simulink model "MAJOR_PROJECT_FINAL"  (R2023b)
settings: Solver=VariableStepAuto  StartTime=0.0  StopTime=inf  FixedStep=1  RelTol=1e-3
libraries: spsRMSLib x8, spsCurrentMeasurementLib x4, spsVoltageMeasurementLib x4, spsPowerLib x4, spsBreakerLib x3, spsSeriesRLCBranchLib x3, spsACVoltageSourceLib x1, spsPLLLib x1, sps_lib x1
settings Model: Creator=bhavikg27  LastModifiedBy=bhavikg27

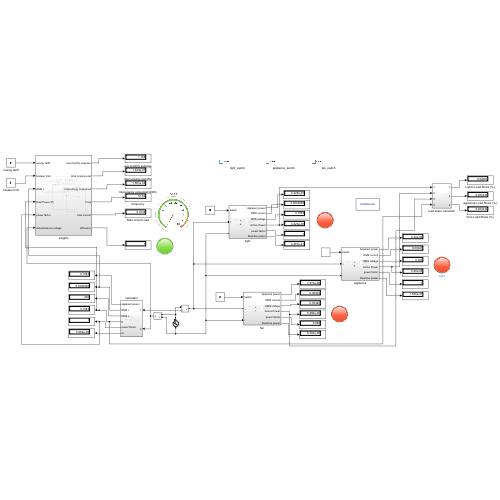
[thumbnail: Simulink's stored preview of the top-level diagram]
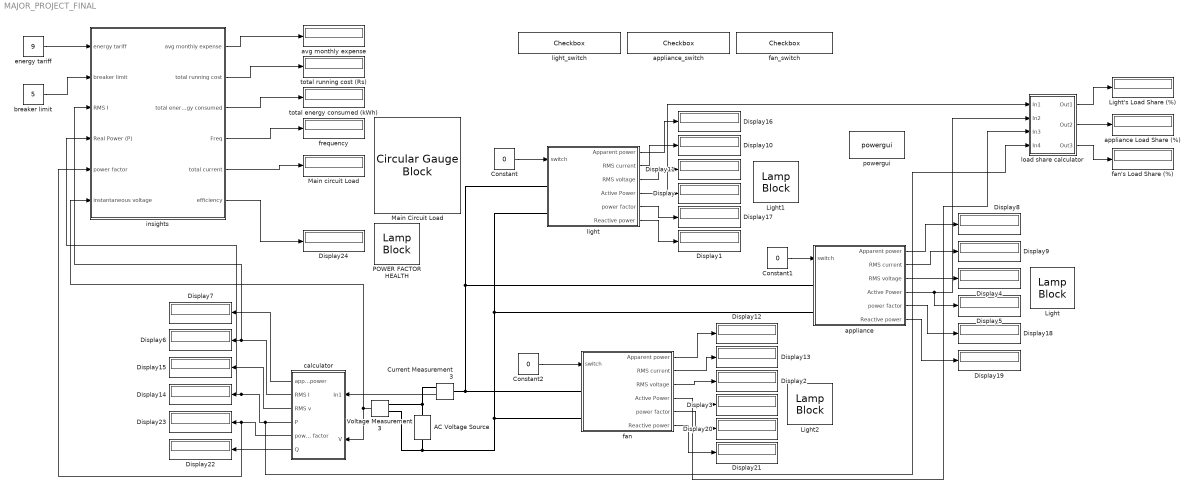
== system MAJOR_PROJECT_FINAL ==
  AC Voltage Source : spsACVoltageSourceLib/AC Voltage Source  Amplitude=325.27  Phase=0  Frequency=50  SampleTime=0  Measurements=None  BusType=swing  Pref=10e3  Qref=0  Qmin=-inf  Qmax=+inf
  Constant : Constant  Value=0
  Constant1 : Constant  Value=0
  Constant2 : Constant  Value=0
  Current Measurement3 : spsCurrentMeasurementLib/Current Measurement  PhasorSimulation=off  OutputType=Complex  PSBequivalent=0
  Display{,1..24} (25 alike) : Display
  Light : LampBlock  LabelPosition=Hide
  Light's Load Share (%) : Display
  Light1 : LampBlock  LabelPosition=Hide
  Light2 : LampBlock  LabelPosition=Hide
  Main Circuit Load : CircularGaugeBlock
  Main circuit Load : Display
  POWER FACTOR HEALTH : LampBlock  LabelPosition=Hide
  Voltage Measurement3 : spsVoltageMeasurementLib/Voltage Measurement  PhasorSimulation=off  OutputType=Complex  PSBequivalent=0
  appliance : Subsystem
  appliance Load Share (%) : Display
  appliance_switch : Checkbox  LabelPosition=Hide  ShowInitialText=on
  avg monthly expense : Display
  breaker limit : Constant  Value=5
  calculator : Subsystem
  energy tariff : Constant  Value=9
  fan : Subsystem
  fan's Load Share (%) : Display
  fan_switch : Checkbox  LabelPosition=Hide  ShowInitialText=on
  frequency : Display
  insights : Subsystem
  light : Subsystem
  light_switch : Checkbox  LabelPosition=Hide  ShowInitialText=on
  load share calculator : Subsystem
  powergui : sps_lib/powergui  Priority=1  SimulationMode=Continuous  SampleTime=50e-6  frequency=60  Iterations=50  frequencyindice=50  Pbase=100e6  ErrMax=1e-4  UnitsV=kV  UnitsW=MW  buscounter=0  FunctionMessages=off  echomessages=off  EnableUseOfTLC=off  CurrentSourceSwitches=off  DisableSnubberDevices=off  DisableRonSwitches=off  DisableVfSwitches=off  DisplayEquations=off  AutomaticDiscreteSolvers=off  SolverType=Tustin/Backward Euler (TBE)  Interpol=off  ExternalGateDelay=off  methode=off  Ts=100  x0status=blocks  SPID=on  SwTol=0  HookPort=off  NonlinearTolerance=1e-4  nMaxIteration=100  ContinueOnMaxIteration=off  RestoreLinks=warning  ResistiveCurrentMeasurement=off  Frange=[0:2:500]  Ylog=off  Xlog=on  ShowGrid=off  save=off  variable=ZData  structure=0  ZoomFFT=off  StartTime=0.0  cycles=1  DisplayStyle=1  fundamental=60  FreqAxis=off  MaxFrequency=1000  frequencyindicesteady=1  RmsSteady=1  display=off
  total energy consumed (kWh) : Display
  total running cost (Rs) : Display
  wires:
  Constant1/1 -> appliance/1(switch)
  Constant2/1 -> fan/1(switch)
  Constant/1 -> light/1(switch)
  light/2(RMS current) -> Display10/1
  light/3(RMS voltage) -> Display11/1
  light/4(Active Power) -> load share calculator/1(In1), Display/1
  light/6(Reactive power) -> Display1/1
  light/1(Apparent power) -> Display16/1
  light/5(power factor) -> Display17/1
  fan/1(Apparent power) -> Display12/1
  fan/3(RMS voltage) -> Display2/1
  fan/4(Active Power) -> load share calculator/3(In3), Display3/1
  fan/6(Reactive power) -> Display21/1
  fan/5(power factor) -> Display20/1
  appliance/1(Apparent power) -> Display8/1
  appliance/2(RMS current) -> Display9/1
  appliance/3(RMS voltage) -> Display4/1
  appliance/4(Active Power) -> load share calculator/2(In2), Display5/1
  appliance/5(power factor) -> Display18/1
  appliance/6(Reactive power) -> Display19/1
  fan/2(RMS current) -> Display13/1
  Voltage Measurement3/1 -> calculator/2(V), insights/6(instantaneous voltage)
  Current Measurement3/1 -> calculator/1(In1)
  calculator/1(apparant power) -> Display7/1
  calculator/2(RMS I) -> insights/3(RMS I), Display6/1
  calculator/3(RMS v) -> Display15/1
  calculator/4(P) -> load share calculator/4(In4), insights/4(Real Power (P)), Display14/1
  calculator/5(power factor) -> insights/5(power factor), Display23/1
  calculator/6(Q) -> Display22/1
  load share calculator/1(Out1) -> Light's Load Share (%)/1
  load share calculator/2(Out2) -> appliance Load Share (%)/1
  load share calculator/3(Out3) -> fan's Load Share (%)/1
  energy tariff/1 -> insights/1(energy tariff)
  breaker limit/1 -> insights/2(breaker limit)
  insights/1(avg monthly expense) -> avg monthly expense/1
  insights/2(total running cost) -> total running cost (Rs)/1
  insights/3(total energy consumed) -> total energy consumed (kWh)/1
  insights/4(Freq) -> frequency/1
  insights/5(total current) -> Main circuit Load/1
  insights/6(efficiency) -> Display24/1
  connections:
  Voltage Measurement3/LConn1 -- AC Voltage Source/LConn1 -- light/LConn2 -- appliance/LConn2 -- fan/LConn2
  Current Measurement3/RConn1 -- Voltage Measurement3/LConn2 -- AC Voltage Source/RConn1
  Current Measurement3/LConn1 -- fan/LConn1 -- light/LConn1 -- appliance/LConn1

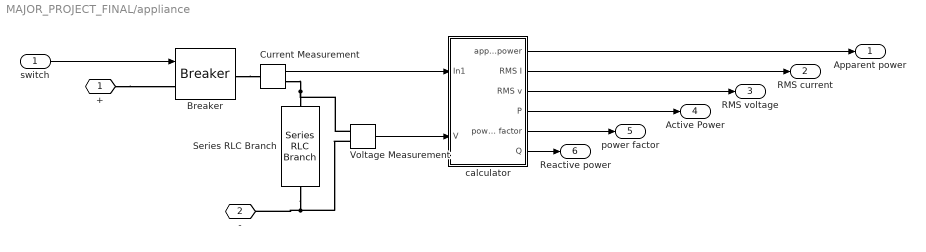
== system MAJOR_PROJECT_FINAL/appliance ==
  switch : Inport
  Breaker : spsBreakerLib/Breaker  InitialState=0  SwitchingTimes="[1/60  5/60]"  External=on  BreakerResistance=0.01  SnubberResistance=1e6  SnubberCapacitance=inf  Measurements=None  MoreParameters=on  NoBreakLoop=off
  Current Measurement : spsCurrentMeasurementLib/Current Measurement  PhasorSimulation=off  OutputType=Complex  PSBequivalent=0
  Series RLC Branch : spsSeriesRLCBranchLib/Series RLC Branch  LConnTagsString=__new0  RConnTagsString=__new0  BranchType=R  Resistance=100  Inductance=1e-3  SetiL0=off  InitialCurrent=0  Capacitance=1e-6  Setx0=off  InitialVoltage=0  Measurements=None
  Voltage Measurement : spsVoltageMeasurementLib/Voltage Measurement  PhasorSimulation=off  OutputType=Complex  PSBequivalent=0
  calculator : Subsystem
  + : PMIOPort  Side=Left
  - : PMIOPort  Port=2  Side=Left
  Apparent power : Outport
  RMS current : Outport  Port=2
  RMS voltage : Outport  Port=3
  Active Power : Outport  Port=4
  power factor : Outport  Port=5
  Reactive power : Outport  Port=6
  wires:
  switch/1 -> Breaker/1
  calculator/5(power factor) -> power factor/1
  calculator/6(Q) -> Reactive power/1
  calculator/4(P) -> Active Power/1
  calculator/2(RMS I) -> RMS current/1
  Voltage Measurement/1 -> calculator/2(V)
  Current Measurement/1 -> calculator/1(In1)
  calculator/1(apparant power) -> Apparent power/1
  calculator/3(RMS v) -> RMS voltage/1
  connections:
  +/RConn1 -- Breaker/LConn1
  Breaker/RConn1 -- Current Measurement/LConn1
  Series RLC Branch/RConn1 -- Voltage Measurement/LConn2 -- -/RConn1
  Current Measurement/RConn1 -- Voltage Measurement/LConn1 -- Series RLC Branch/LConn1

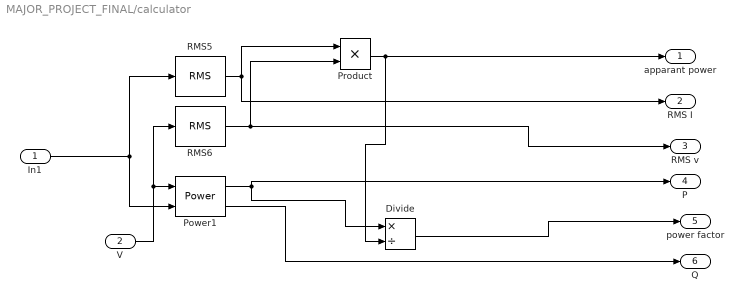
== system MAJOR_PROJECT_FINAL/calculator ==
  In1 : Inport
  V : Inport  Port=2
  Divide : Product  Inputs=*/
  Power1 : spsPowerLib/Power  Freq=50  Vinit=[1, 0]  Iinit=[1, 0]  Ts=0
  Product : Product
  RMS5 : spsRMSLib/RMS  TrueRMS=on  Freq=50  RMSInit=120  Ts=0
  RMS6 : spsRMSLib/RMS  TrueRMS=on  Freq=50  RMSInit=120  Ts=0
  apparant power : Outport
  RMS I : Outport  Port=2
  RMS v : Outport  Port=3
  P : Outport  Port=4
  power factor : Outport  Port=5
  Q : Outport  Port=6
  wires:
  V/1 -> RMS6/1, Power1/1
  In1/1 -> Power1/2, RMS5/1
  RMS5/1 -> RMS I/1, Product/1
  RMS6/1 -> RMS v/1, Product/2
  Power1/1 -> P/1, Divide/1
  Product/1 -> apparant power/1, Divide/2
  Divide/1 -> power factor/1
  Power1/2 -> Q/1

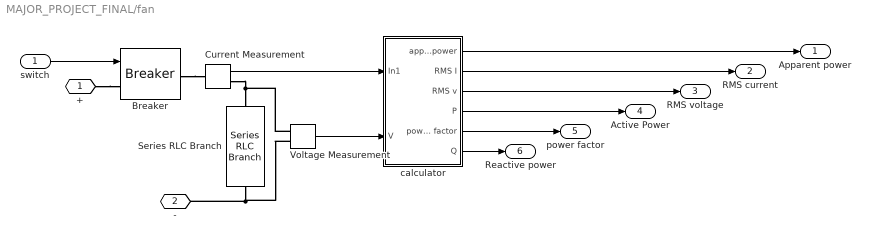
== system MAJOR_PROJECT_FINAL/fan ==
  switch : Inport
  Breaker : spsBreakerLib/Breaker  InitialState=0  SwitchingTimes="[1/60  5/60]"  External=on  BreakerResistance=0.01  SnubberResistance=1e6  SnubberCapacitance=inf  Measurements=None  MoreParameters=on  NoBreakLoop=off
  Current Measurement : spsCurrentMeasurementLib/Current Measurement  PhasorSimulation=off  OutputType=Complex  PSBequivalent=0
  Series RLC Branch : spsSeriesRLCBranchLib/Series RLC Branch  LConnTagsString=__new0  RConnTagsString=__new0  BranchType=RL  Resistance=100  Inductance=0.3  SetiL0=off  InitialCurrent=0  Capacitance=1e-6  Setx0=off  InitialVoltage=0  Measurements=None
  Voltage Measurement : spsVoltageMeasurementLib/Voltage Measurement  PhasorSimulation=off  OutputType=Complex  PSBequivalent=0
  calculator : Subsystem
  + : PMIOPort  Side=Left
  - : PMIOPort  Port=2  Side=Left
  Apparent power : Outport
  RMS current : Outport  Port=2
  RMS voltage : Outport  Port=3
  Active Power : Outport  Port=4
  power factor : Outport  Port=5
  Reactive power : Outport  Port=6
  wires:
  switch/1 -> Breaker/1
  calculator/5(power factor) -> power factor/1
  calculator/6(Q) -> Reactive power/1
  calculator/4(P) -> Active Power/1
  calculator/2(RMS I) -> RMS current/1
  Voltage Measurement/1 -> calculator/2(V)
  Current Measurement/1 -> calculator/1(In1)
  calculator/1(apparant power) -> Apparent power/1
  calculator/3(RMS v) -> RMS voltage/1
  connections:
  +/RConn1 -- Breaker/LConn1
  Breaker/RConn1 -- Current Measurement/LConn1
  Series RLC Branch/RConn1 -- -/RConn1 -- Voltage Measurement/LConn2
  Current Measurement/RConn1 -- Voltage Measurement/LConn1 -- Series RLC Branch/LConn1

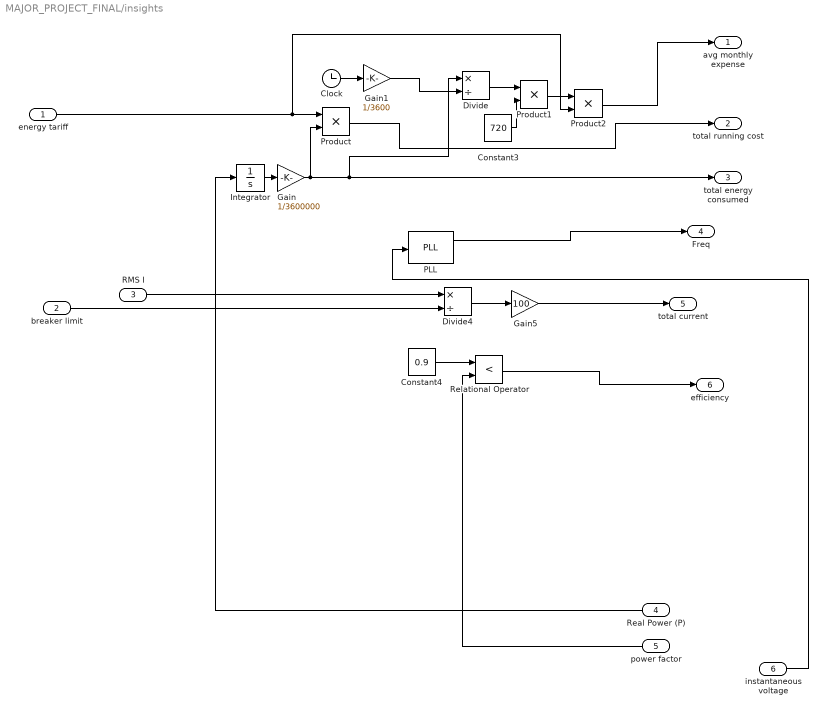
== system MAJOR_PROJECT_FINAL/insights ==
  energy tariff : Inport
  breaker limit : Inport  Port=2
  RMS I : Inport  Port=3
  Real Power (P) : Inport  Port=4
  power factor : Inport  Port=5
  instantaneous voltage : Inport  Port=6
  Clock : Clock
  Constant3 : Constant  Value=720
  Constant4 : Constant  Value=0.9
  Divide : Product  Inputs=*/
  Divide4 : Product  Inputs=*/
  Gain : Gain  Gain=1/3600000
  Gain1 : Gain  Gain=1/3600
  Gain5 : Gain  Gain=100
  Integrator : Integrator
  PLL : spsPLLLib/PLL  Fmin=45  Par_Init=[0, 60]  ParK=[180, 3200, 1]  TcD=1e-4  MaxRateChangeFreq=12  FilterCutOffFreq=25  Ts=0  AGC=on
      settings: LibrarySourceBlock=sps_lib/Control/PLL
  Product : Product
  Product1 : Product
  Product2 : Product
  Relational Operator : RelationalOperator  Operator=<  OutDataTypeStr=boolean  RndMeth=Simplest  InputSameDT=off
  avg monthly expense : Outport
  total running cost : Outport  Port=2
  total energy consumed : Outport  Port=3
  Freq : Outport  Port=4
  total current : Outport  Port=5
  efficiency : Outport  Port=6
  wires:
  Gain/1 -> total energy consumed/1, Divide/1, Product/2
  Divide/1 -> Product1/1
  energy tariff/1 -> Product/1, Product2/2
  Divide4/1 -> Gain5/1
  Integrator/1 -> Gain/1
  Real Power (P)/1 -> Integrator/1
  Clock/1 -> Gain1/1
  Product1/1 -> Product2/1
  Gain1/1 -> Divide/2
  Relational Operator/1 -> efficiency/1
  Constant3/1 -> Product1/2
  Constant4/1 -> Relational Operator/1
  Product/1 -> total running cost/1
  Product2/1 -> avg monthly expense/1
  Gain5/1 -> total current/1
  breaker limit/1 -> Divide4/2
  instantaneous voltage/1 -> PLL/1
  PLL/1 -> Freq/1
  RMS I/1 -> Divide4/1
  power factor/1 -> Relational Operator/2

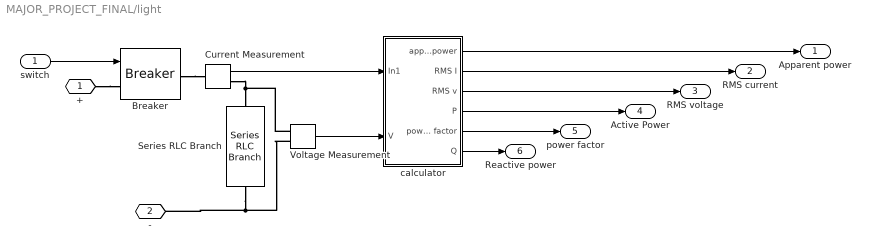
== system MAJOR_PROJECT_FINAL/light ==
  switch : Inport
  Breaker : spsBreakerLib/Breaker  InitialState=0  SwitchingTimes="[1/60  5/60]"  External=on  BreakerResistance=0.01  SnubberResistance=1e6  SnubberCapacitance=inf  Measurements=None  MoreParameters=on  NoBreakLoop=off
  Current Measurement : spsCurrentMeasurementLib/Current Measurement  PhasorSimulation=off  OutputType=Complex  PSBequivalent=0
  Series RLC Branch : spsSeriesRLCBranchLib/Series RLC Branch  LConnTagsString=__new0  RConnTagsString=__new0  BranchType=R  Resistance=800  Inductance=1e-3  SetiL0=off  InitialCurrent=0  Capacitance=1e-6  Setx0=off  InitialVoltage=0  Measurements=None
  Voltage Measurement : spsVoltageMeasurementLib/Voltage Measurement  PhasorSimulation=off  OutputType=Complex  PSBequivalent=0
  calculator : Subsystem
  + : PMIOPort  Side=Left
  - : PMIOPort  Port=2  Side=Left
  Apparent power : Outport
  RMS current : Outport  Port=2
  RMS voltage : Outport  Port=3
  Active Power : Outport  Port=4
  power factor : Outport  Port=5
  Reactive power : Outport  Port=6
  wires:
  switch/1 -> Breaker/1
  Current Measurement/1 -> calculator/1(In1)
  Voltage Measurement/1 -> calculator/2(V)
  calculator/1(apparant power) -> Apparent power/1
  calculator/2(RMS I) -> RMS current/1
  calculator/3(RMS v) -> RMS voltage/1
  calculator/4(P) -> Active Power/1
  calculator/5(power factor) -> power factor/1
  calculator/6(Q) -> Reactive power/1
  connections:
  +/RConn1 -- Breaker/LConn1
  Breaker/RConn1 -- Current Measurement/LConn1
  Series RLC Branch/RConn1 -- -/RConn1 -- Voltage Measurement/LConn2
  Current Measurement/RConn1 -- Voltage Measurement/LConn1 -- Series RLC Branch/LConn1

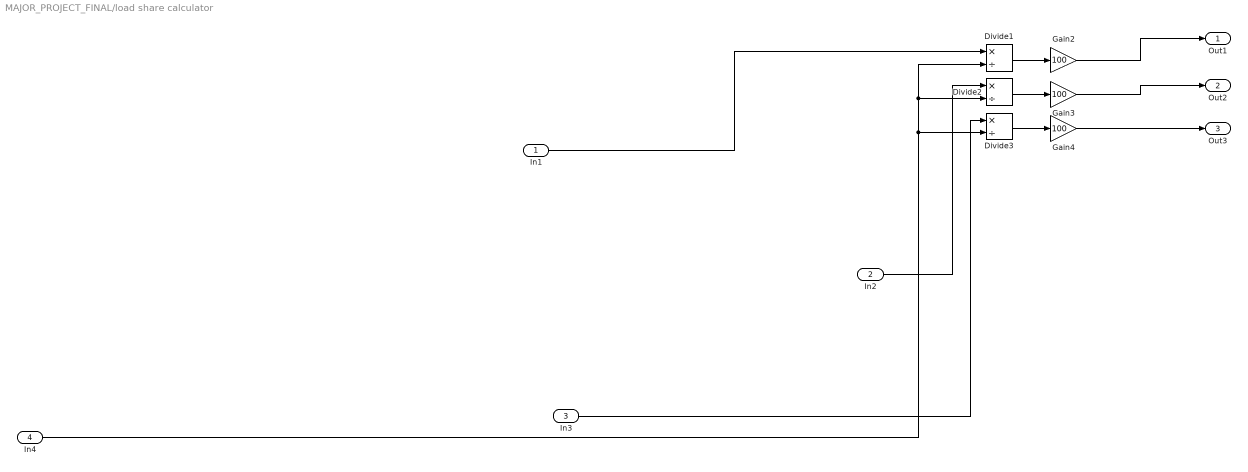
== system MAJOR_PROJECT_FINAL/load share calculator ==
  In1 : Inport
  In2 : Inport  Port=2
  In3 : Inport  Port=3
  In4 : Inport  Port=4
  Divide1 : Product  Inputs=*/
  Divide2 : Product  Inputs=*/
  Divide3 : Product  Inputs=*/
  Gain2 : Gain  Gain=100
  Gain3 : Gain  Gain=100
  Gain4 : Gain  Gain=100
  Out1 : Outport
  Out2 : Outport  Port=2
  Out3 : Outport  Port=3
  wires:
  Divide2/1 -> Gain3/1
  Divide1/1 -> Gain2/1
  Gain2/1 -> Out1/1
  In4/1 -> Divide3/2, Divide2/2, Divide1/2
  Divide3/1 -> Gain4/1
  In1/1 -> Divide1/1
  Gain3/1 -> Out2/1
  In2/1 -> Divide2/1
  In3/1 -> Divide3/1
  Gain4/1 -> Out3/1

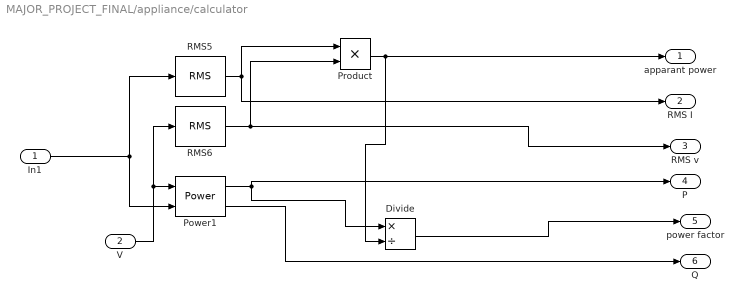
== system MAJOR_PROJECT_FINAL/appliance/calculator ==
  In1 : Inport
  V : Inport  Port=2
  Divide : Product  Inputs=*/
  Power1 : spsPowerLib/Power  Freq=50  Vinit=[1, 0]  Iinit=[1, 0]  Ts=0
  Product : Product
  RMS5 : spsRMSLib/RMS  TrueRMS=on  Freq=50  RMSInit=120  Ts=0
  RMS6 : spsRMSLib/RMS  TrueRMS=on  Freq=50  RMSInit=120  Ts=0
  apparant power : Outport
  RMS I : Outport  Port=2
  RMS v : Outport  Port=3
  P : Outport  Port=4
  power factor : Outport  Port=5
  Q : Outport  Port=6
  wires:
  V/1 -> RMS6/1, Power1/1
  In1/1 -> Power1/2, RMS5/1
  RMS5/1 -> RMS I/1, Product/1
  RMS6/1 -> RMS v/1, Product/2
  Power1/1 -> P/1, Divide/1
  Product/1 -> apparant power/1, Divide/2
  Divide/1 -> power factor/1
  Power1/2 -> Q/1

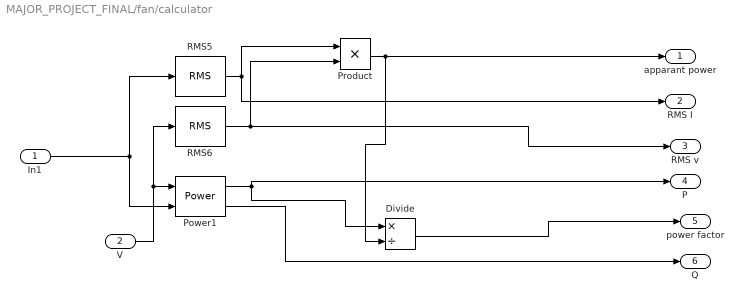
== system MAJOR_PROJECT_FINAL/fan/calculator ==
  In1 : Inport
  V : Inport  Port=2
  Divide : Product  Inputs=*/
  Power1 : spsPowerLib/Power  Freq=50  Vinit=[1, 0]  Iinit=[1, 0]  Ts=0
  Product : Product
  RMS5 : spsRMSLib/RMS  TrueRMS=on  Freq=50  RMSInit=120  Ts=0
  RMS6 : spsRMSLib/RMS  TrueRMS=on  Freq=50  RMSInit=120  Ts=0
  apparant power : Outport
  RMS I : Outport  Port=2
  RMS v : Outport  Port=3
  P : Outport  Port=4
  power factor : Outport  Port=5
  Q : Outport  Port=6
  wires:
  V/1 -> RMS6/1, Power1/1
  In1/1 -> Power1/2, RMS5/1
  RMS5/1 -> RMS I/1, Product/1
  RMS6/1 -> RMS v/1, Product/2
  Power1/1 -> P/1, Divide/1
  Product/1 -> apparant power/1, Divide/2
  Divide/1 -> power factor/1
  Power1/2 -> Q/1

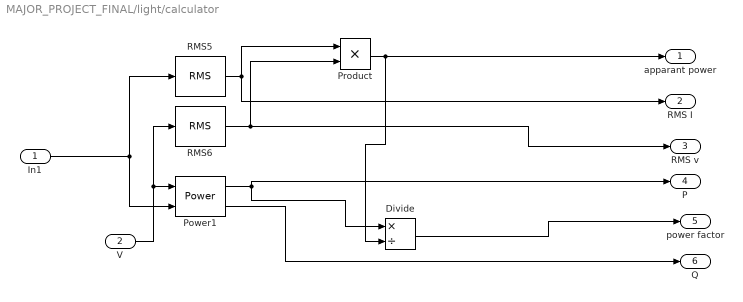
== system MAJOR_PROJECT_FINAL/light/calculator ==
  In1 : Inport
  V : Inport  Port=2
  Divide : Product  Inputs=*/
  Power1 : spsPowerLib/Power  Freq=50  Vinit=[1, 0]  Iinit=[1, 0]  Ts=0
  Product : Product
  RMS5 : spsRMSLib/RMS  TrueRMS=on  Freq=50  RMSInit=120  Ts=0
  RMS6 : spsRMSLib/RMS  TrueRMS=on  Freq=50  RMSInit=120  Ts=0
  apparant power : Outport
  RMS I : Outport  Port=2
  RMS v : Outport  Port=3
  P : Outport  Port=4
  power factor : Outport  Port=5
  Q : Outport  Port=6
  wires:
  V/1 -> RMS6/1, Power1/1
  In1/1 -> Power1/2, RMS5/1
  RMS5/1 -> RMS I/1, Product/1
  RMS6/1 -> RMS v/1, Product/2
  Power1/1 -> P/1, Divide/1
  Product/1 -> apparant power/1, Divide/2
  Divide/1 -> power factor/1
  Power1/2 -> Q/1
